simulink subsystem "OneAxleTrailer"  (R2023a)
settings: Solver=VariableStepAuto  StartTime=0.0  StopTime=10.0  RelTol=1e-3
undefined symbols (not defined in the file): PlntTraCGHgtAxl, PlntTraDstCGMiddleAxl, PlntTraHtchCxy, PlntTraHtchCz, PlntTraHtchF0z, PlntTraHtchKxy, PlntTraHtchKz, PlntTraInitLatPos, PlntTraInitLatVel, PlntTraInitLongPos, PlntTraInitLongVel, PlntTraInitPitchAng, PlntTraInitPitchRate, PlntTraInitRollAng, PlntTraInitRollRate, PlntTraInitVertPos, PlntTraInitVertVel, PlntTraInitYawAng, PlntTraInitYawRate, PlntTraMass, PlntTraNumWhlFrntAxl, PlntTraPitchMomentInertia, PlntTraRollMomentInertia, PlntTraTrckWdth, PlntTraYawMomentInertia
libraries: autolibutils x7, sharedtransform x4, vehdynlibeom x2, vehdynlibsuspension x1, matrix_library x1
(part 1 of 2)
settings Model: ModifiedByFormat=The MathWorks, Inc.  Creator=The MathWorks, Inc.  LastModifiedBy=The MathWorks, Inc.
settings SolverCC: MaxZcPerStep=1
settings OptimizationCC: ReuseModelBlockBuffer=off
settings DebuggingCC: UnconnectedInputMsg=warning  UnconnectedOutputMsg=warning  UnconnectedLineMsg=warning
settings ModelReferenceCC: EnableRefExpFcnMdlSchedulingChecks=on
settings RTWCC: DLArmComputeVersion=19.05

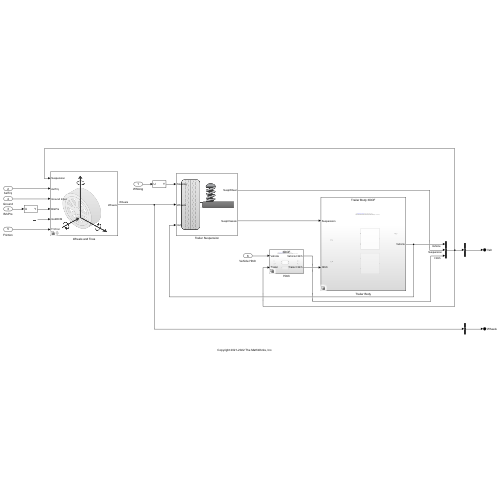
[thumbnail: Simulink's stored preview of the top-level diagram]
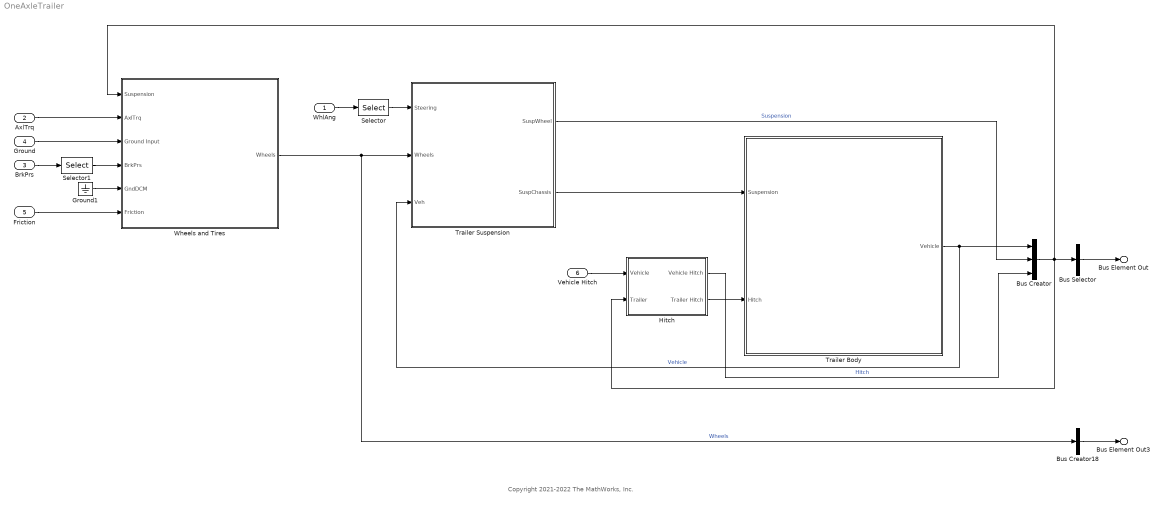
== system OneAxleTrailer ==
  note: Copyright 2021-2022 The MathWorks, Inc.
  WhlAng : Inport
  AxlTrq : Inport  Port=2
  BrkPrs : Inport  Port=3
  Ground : Inport  Port=4
  Friction : Inport  Port=5
  Vehicle Hitch : Inport  Port=6
  Bus Creator : BusCreator  Inputs=3
  Bus Creator18 : BusCreator  Inputs=1
  Bus Selector : BusSelector  OutputSignals=Vehicle.InertFrm,Vehicle.BdyFrm,Hitch  OutputAsBus=on
  Ground1 : Ground
  Hitch : Subsystem  Variant=on  VariantControlMode=label  LabelModeActiveChoice=0
  Selector : Selector  IndexOptions=Index vector (dialog)  Indices=[1 2]  OutputSizes=1
  Selector1 : Selector  IndexOptions=Index vector (dialog)  Indices=[1 2]  OutputSizes=1
  Trailer Body : Subsystem  Variant=on  VariantControlMode=label  LabelModeActiveChoice=0
  Trailer Suspension : Subsystem
      mask Display: image('suspsacoil.png')
  Wheels and Tires : Subsystem  Variant=on  VariantControlMode=label  VariantControl=Choice  LabelModeActiveChoice=MF Tires Longitudinal and Lateral
      mask Display: image('wheel3dof.png')
  Bus Element Out : Outport  PortName=Veh
  Bus Element Out3 : Outport  Port=2  PortName=Wheels
  wires:
  Trailer Suspension/1(SuspWheel) -> Bus Creator/2  "Suspension"
  Trailer Suspension/2(SuspChassis) -> Trailer Body/1(Suspension)
  Bus Creator18/1 -> Bus Element Out3/1
  Vehicle Hitch/1 -> Hitch/1(Vehicle)
  Bus Selector/1 -> Bus Element Out/1
  Hitch/1(Vehicle Hitch) -> Bus Creator/3  "Hitch"
  AxlTrq/1 -> Wheels and Tires/2(AxlTrq)
  Bus Creator/1 -> Hitch/2(Trailer), Bus Selector/1, Wheels and Tires/1(Suspension)
  Wheels and Tires/1(Wheels) -> Bus Creator18/1, Trailer Suspension/2(Wheels)  "Wheels"
  BrkPrs/1 -> Selector1/1
  WhlAng/1 -> Selector/1
  Friction/1 -> Wheels and Tires/6(Friction)
  Trailer Body/1(Vehicle) -> Bus Creator/1, Trailer Suspension/3(Veh)  "Vehicle"
  Hitch/2(Trailer Hitch) -> Trailer Body/2(Hitch)
  Selector/1 -> Trailer Suspension/1(Steering)
  Selector1/1 -> Wheels and Tires/4(BrkPrs)
  Ground/1 -> Wheels and Tires/3(Ground Input)
  Ground1/1 -> Wheels and Tires/5(GndDCM)

== system OneAxleTrailer/Hitch ==
  note: 1) Add Subsystem or Model blocks as valid variant choices.
      | 2) You cannot connect blocks at this level. At simulation, connectivity is automatically
      | determined, based on the active variant and port name matching.
  Vehicle : Inport
  Trailer : Inport  Port=2
  3DOF : Subsystem  VariantControl=0
  6DOF : Subsystem  VariantControl=1
  Vehicle Hitch : Outport
  Trailer Hitch : Outport  Port=2

== system OneAxleTrailer/Trailer Body ==
  note: 1) Add Subsystem or Model blocks as valid variant choices.
      | 2) You cannot connect blocks at this level. At simulation, connectivity is automatically
      | determined, based on the active variant and port name matching.
  Suspension : Inport
  Hitch : Inport  Port=2
  Trailer Body 3DOF : Subsystem  VariantControl=0
  Trailer Body 6DOF : Subsystem  VariantControl=1
  Vehicle : Outport

== system OneAxleTrailer/Trailer Suspension ==
  Steering : Inport
  Wheels : Inport  Port=2
  Veh : Inport  Port=3
  Bus Creator : BusCreator  Inputs=2
  Solid Axle Suspension : Subsystem  VariantControl=MacPherson Front Suspension Solid Axle Rear Suspension
      mask Display: image('suspsacoil.png');
  Susp2Wheel : Subsystem
  Wheel2Susp : Subsystem
  SuspWheel : Outport
  SuspChassis : Outport  Port=2
  wires:
  Solid Axle Suspension/1(Suspension) -> Susp2Wheel/1(Susp), Bus Creator/1  "SuspChassis"
  Wheel2Susp/1(Wheels2Susp) -> Solid Axle Suspension/3(Wheels), Susp2Wheel/2(WheelSusp)
  Susp2Wheel/1(SuspWheel) -> SuspWheel/1, Bus Creator/2, Wheel2Susp/3(SuspWheel)  "SuspWheel"
  Wheels/1 -> Wheel2Susp/2(Wheels)
  Bus Creator/1 -> SuspChassis/1
  Veh/1 -> Wheel2Susp/1(Veh), Solid Axle Suspension/2(Vehicle)
  Steering/1 -> Solid Axle Suspension/1(Steer)

== system OneAxleTrailer/Wheels and Tires ==
  Suspension : Inport
  AxlTrq : Inport  Port=2
  Ground Input : Inport  Port=3
  BrkPrs : Inport  Port=4
  GndDCM : Inport  Port=5
  Friction : Inport  Port=6
  Combined Slip Tires Longitudinal : Subsystem  VariantControl=Combined Slip Tires Longitudinal  ReferencedSubsystem=CombinedSlipTrailerTiresLongitudinal
  Fiala Tires Longitudinal and Lateral : Subsystem  VariantControl=Fiala Tires Longitudinal and Lateral  ReferencedSubsystem=FialaTrailerTires
  MF Tires Longitudinal : Subsystem  VariantControl=MF Tires Longitudinal  ReferencedSubsystem=MFTrailerTiresLongitudinal
  MF Tires Longitudinal and Lateral : Subsystem  VariantControl=MF Tires Longitudinal and Lateral  ReferencedSubsystem=MFTrailerTires
  Wheels : Outport

== system OneAxleTrailer/Hitch/3DOF ==
  Vehicle : Inport
  Trailer : Inport  Port=2
  Bus Selector : BusSelector  OutputSignals=InertFrm.Hitch.Disp.X,InertFrm.Hitch.Disp.Y,InertFrm.Cg.Ang.psi,InertFrm.Hitch.Vel.Xdot,InertFrm.Hitch.Vel.Ydot
  Bus Selector1 : BusSelector  OutputSignals=Vehicle.InertFrm.HitchF.Disp.X,Vehicle.InertFrm.HitchF.Disp.Y,Vehicle.InertFrm.Cg.Ang.psi,Vehicle.BdyFrm.Forces.HitchF.Fz,Vehicle.InertFrm.HitchF.Vel.Xdot,Vehicle.InertFrm.HitchF.Vel.Ydot
  Mux : Mux  Inputs=6
  Mux1 : Mux  Inputs=6
  Subsystem3 : Subsystem
  Vehicle Hitch : Outport
  Trailer Hitch : Outport  Port=2
  wires:
  Subsystem3/6(Vehicle Mhz) -> Mux1/6
  Subsystem3/5(Vehicle Mhy) -> Mux1/5
  Subsystem3/4(Vehicle Mhx) -> Mux1/4
  Subsystem3/12(Trailer Mhz) -> Mux/6
  Subsystem3/11(Trailer Mhy) -> Mux/5
  Subsystem3/10(Trailer Mhx) -> Mux/4
  Bus Selector1/6 -> Subsystem3/11(Trailer Ydot)  "<Ydot>"
  Bus Selector1/5 -> Subsystem3/10(Trailer Xdot)  "<Xdot>"
  Bus Selector/5 -> Subsystem3/5(Vehicle Ydot)  "<Ydot>"
  Bus Selector/4 -> Subsystem3/4(Vehicle Xdot)  "<Xdot>"
  Subsystem3/8(Trailer Fy) -> Mux/2
  Subsystem3/7(Trailer Fx) -> Mux/1
  Subsystem3/3(Vehicle Fz) -> Mux1/3
  Subsystem3/2(Vehicle Fy) -> Mux1/2
  Subsystem3/1(Vehicle Fx) -> Mux1/1
  Bus Selector1/3 -> Subsystem3/8(Trailer psi)  "<psi>"
  Bus Selector1/4 -> Subsystem3/9(Trailer Fz)  "<Fz>"
  Bus Selector1/2 -> Subsystem3/7(Trailer Y)  "<Y>"
  Bus Selector1/1 -> Subsystem3/6(Trailer X)  "<X>"
  Bus Selector/3 -> Subsystem3/3(Vehicle psi)  "<psi>"
  Bus Selector/2 -> Subsystem3/2(Vehicle Y)  "<Y>"
  Bus Selector/1 -> Subsystem3/1(Vehicle X)  "<X>"
  Trailer/1 -> Bus Selector1/1
  Mux/1 -> Trailer Hitch/1
  Vehicle/1 -> Bus Selector/1
  Mux1/1 -> Vehicle Hitch/1
  Subsystem3/9(Trailer FzOut) -> Mux/3

== system OneAxleTrailer/Hitch/6DOF ==
  Vehicle : Inport
  Trailer : Inport  Port=2
  Bus Selector : BusSelector  OutputSignals=InertFrm.Hitch.Disp.X,InertFrm.Hitch.Disp.Y,InertFrm.Hitch.Disp.Z,InertFrm.Hitch.Vel.Xdot,InertFrm.Hitch.Vel.Ydot,InertFrm.Hitch.Vel.Zdot,InertFrm.Cg.Ang.psi
  Bus Selector1 : BusSelector  OutputSignals=Vehicle.InertFrm.HitchF.Disp.X,Vehicle.InertFrm.HitchF.Disp.Y,Vehicle.InertFrm.HitchF.Disp.Z,Vehicle.InertFrm.HitchF.Vel.Xdot,Vehicle.InertFrm.HitchF.Vel.Ydot,Vehicle.InertFrm.HitchF.Vel.Zdot,Vehicle.InertFrm.Cg.Ang.psi
  Mux : Mux  Inputs=6
  Mux1 : Mux  Inputs=6
  Subsystem3 : Subsystem
  Vehicle Hitch : Outport
  Trailer Hitch : Outport  Port=2
  wires:
  Subsystem3/6(Vehicle Mhz) -> Mux1/6
  Subsystem3/5(Vehicle Mhy) -> Mux1/5
  Subsystem3/4(Vehicle Mhx) -> Mux1/4
  Subsystem3/12(Trailer Mhz) -> Mux/6
  Subsystem3/11(Trailer Mhy) -> Mux/5
  Subsystem3/10(Trailer Mhx) -> Mux/4
  Bus Selector/5 -> Subsystem3/5(Vehicle Ydot)  "<Ydot>"
  Bus Selector/4 -> Subsystem3/4(Vehicle Xdot)  "<Xdot>"
  Bus Selector1/4 -> Subsystem3/11(Trailer Xdot)  "<Xdot>"
  Bus Selector1/5 -> Subsystem3/12(Trailer Ydot)  "<Ydot>"
  Bus Selector1/6 -> Subsystem3/13(Trailer Zdot)  "<Zdot>"
  Bus Selector/6 -> Subsystem3/6(Vehicle Zdot)  "<Zdot>"
  Bus Selector/3 -> Subsystem3/3(Vehicle Z)  "<Z>"
  Bus Selector1/3 -> Subsystem3/10(Trailer Z)  "<Z>"
  Subsystem3/8(Trailer Fy) -> Mux/2
  Subsystem3/7(Trailer Fx) -> Mux/1
  Subsystem3/3(Vehicle Fz) -> Mux1/3
  Subsystem3/2(Vehicle Fy) -> Mux1/2
  Subsystem3/1(Vehicle Fx) -> Mux1/1
  Bus Selector1/7 -> Subsystem3/14(Trailer psi)  "<psi>"
  Bus Selector1/2 -> Subsystem3/9(Trailer Y)  "<Y>"
  Bus Selector1/1 -> Subsystem3/8(Trailer X)  "<X>"
  Bus Selector/7 -> Subsystem3/7(Vehicle psi)  "<psi>"
  Bus Selector/2 -> Subsystem3/2(Vehicle Y)  "<Y>"
  Bus Selector/1 -> Subsystem3/1(Vehicle X)  "<X>"
  Trailer/1 -> Bus Selector1/1
  Mux/1 -> Trailer Hitch/1
  Vehicle/1 -> Bus Selector/1
  Mux1/1 -> Vehicle Hitch/1
  Subsystem3/9(Trailer Fz) -> Mux/3

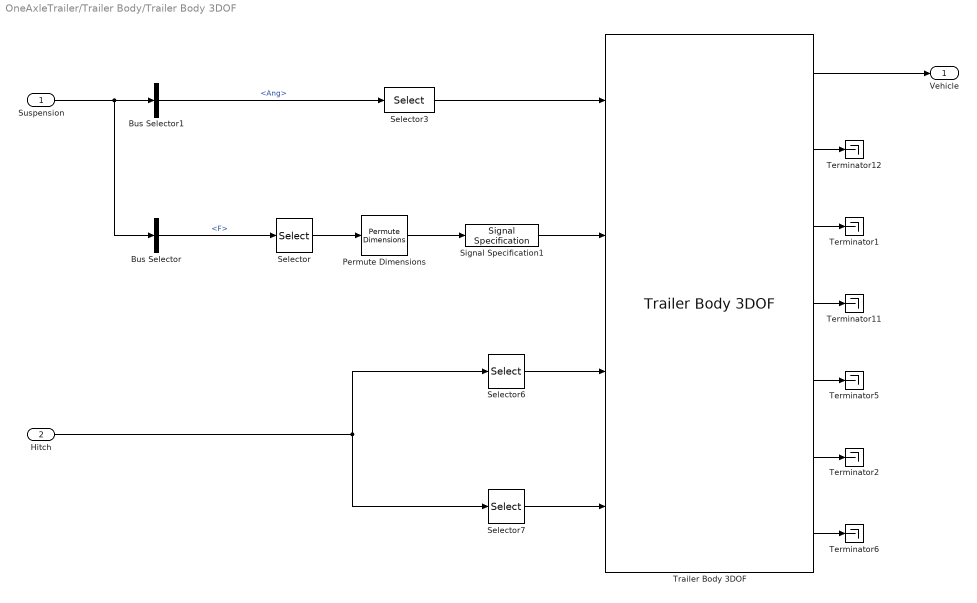
== system OneAxleTrailer/Trailer Body/Trailer Body 3DOF ==
  Suspension : Inport
  Hitch : Inport  Port=2
  Bus Selector : BusSelector  OutputSignals=SuspChassis.Veh.F
  Bus Selector1 : BusSelector  OutputSignals=SuspChassis.Whl.Ang
  Permute Dimensions : PermuteDimensions
  Selector : Selector  NumberOfDimensions=2  InputPortWidth=3  IndexOptions=Index vector (dialog),Index vector (dialog)  Indices=[1 2],[1 2]  OutputSizes=1,1
  Selector3 : Selector  NumberOfDimensions=2  InputPortWidth=6  IndexOptions=Index vector (dialog),Index vector (dialog)  Indices=3,[1 2]  OutputSizes=1,1
  Selector6 : Selector  InputPortWidth=6  IndexOptions=Index vector (dialog)  Indices=[1 2 3]  OutputSizes=1
  Selector7 : Selector  InputPortWidth=6  IndexOptions=Index vector (dialog)  Indices=[4 5 6]  OutputSizes=1
  Signal Specification1 : SignalSpecification  Unit=N
  Terminator{1..2,5..6,11..12} (6 alike) : Terminator
  Trailer Body 3DOF : vehdynlibeom/Trailer Body 3DOF  trackMode=Dual 1-axle  inputMode=External forces  frontSteerMode=on  middleSteerMode=off  rearSteerMode=off  windMode=off  muMode=off  extFMode=off  extMMode=off  FhtchFMode=on  FhtchMMode=on  RhtchFMode=off  RhtchMMode=off  extXo=off  extpsio=off  extxdoto=off  extro=off  extYo=off  extTamb=off  extydoto=off  aMode=2  NF=PlntTraNumWhlFrntAxl  NM=PlntTraNumWhlMiddleAxl  NR=PlntTraNumWhlRearAxl  m=PlntTraMass  a=PlntTraDstCGFrntAxl  b=PlntTraDstCGMiddleAxl  c=PlntTraDstCGRearAxl  h=PlntTraCGHgtAxl  dh_f=PlntTraHtchDstFrnt  hh_f=PlntTraHtchHgtAxlFrnt  dh_r=7.5  hh_r=0.6  X_o=PlntTraInitLongPos  xdot_o=PlntTraInitLongVel  Lcpm=4.5  CalphaMode=off  sigmaMode=on  d=0  hl_f=0  hl_r=0  w_f=PlntTraTrckWdth  w_m=PlntTraTrckWdth  w_r=PlntTraTrckWdth  Cy_f=12e3  Cy_m=11e3  Cy_r=11e3  sigma_f=.1  sigma_m=.1  sigma_r=.1  alpha_f_brk=[-.1 .1]  Cy_f_data=[-9e3 9e3]  alpha_m_brk=[-.1 .1]  Cy_m_data=[-9e3 9e3]  alpha_r_brk=[-.1 .1]  Cy_r_data=[-9e3 9e3]  Y_o=PlntTraInitLatPos  ydot_o=PlntTraInitLatVel  Izz=PlntTraYawMomentInertia  psi_o=PlntTraInitYawAng  r_o=PlntTraInitYawRate  Af=PlntTraAeroFrntArea  Cd=PlntTraAeroDragCff  Cl=PlntTraAeroLiftCff  Cpm=PlntTraAeroPitchCff  beta_w=[0:0.01:0.3]  Cs=[0:0.03:0.9]*0  Cym=[0:0.01:0.3]*0  Pabs=101325  Tair=273  g=9.81  mu=1  xdot_tol=.01  Fznom=5000  Fxtire_sat=7e4  Fytire_sat=7e4  longOff=0  latOff=0  vertOff=0  wrapAng=off
  Vehicle : Outport
  wires:
  Selector7/1 -> Trailer Body 3DOF/4
  Hitch/1 -> Selector6/1, Selector7/1
  Selector6/1 -> Trailer Body 3DOF/3
  Trailer Body 3DOF/4 -> Terminator11/1
  Bus Selector/1 -> Selector/1  "<F>"
  Trailer Body 3DOF/1 -> Vehicle/1
  Selector/1 -> Permute Dimensions/1
  Permute Dimensions/1 -> Signal Specification1/1
  Trailer Body 3DOF/5 -> Terminator5/1
  Selector3/1 -> Trailer Body 3DOF/1
  Signal Specification1/1 -> Trailer Body 3DOF/2
  Bus Selector1/1 -> Selector3/1  "<Ang>"
  Trailer Body 3DOF/3 -> Terminator1/1
  Trailer Body 3DOF/2 -> Terminator12/1
  Trailer Body 3DOF/7 -> Terminator6/1
  Trailer Body 3DOF/6 -> Terminator2/1
  Suspension/1 -> Bus Selector1/1, Bus Selector/1

== system OneAxleTrailer/Trailer Body/Trailer Body 6DOF ==
  Suspension : Inport
  Hitch : Inport  Port=2
  Bus Selector3 : BusSelector  OutputSignals=SuspChassis.Veh.F,SuspChassis.Veh.M
  Constant1 : Constant  Value=zeros(3,1)  SampleTime=-1
  Constant2 : Constant  Value=zeros(3,1)  SampleTime=-1
  Constant3 : Constant  Value=zeros(3,1)  SampleTime=-1
  Selector6 : Selector  InputPortWidth=6  IndexOptions=Index vector (dialog)  Indices=[1 2 3]  OutputSizes=1
  Selector7 : Selector  InputPortWidth=6  IndexOptions=Index vector (dialog)  Indices=[4 5 6]  OutputSizes=1
  Terminator{,1..5} (6 alike) : Terminator
  Trailer Body 6DOF : vehdynlibeom/Trailer Body 6DOF  axleMode=1  extPos=on  extVel=on  extEuler=on  extRotRate=on  htchFMode_f=on  htchMMode_f=on  htchFMode_r=off  htchMMode_r=off  m=PlntTraMass  a=PlntTraDstCGFrntAxl  b=PlntTraDstCGMiddleAxl  c=PlntTraDstCGRearAxl  d=0  h=PlntTraCGHgtAxl  dh_f=PlntTraHtchDstFrnt  hl_f=0  hh_f=PlntTraHtchHgtAxlFrnt  dh_r=1  hl_r=0  hh_r=0.1  Xe_o=[PlntTraInitLongPos,PlntTraInitLatPos,PlntTraInitVertPos]  xbdot_o=[PlntTraInitLongVel,PlntTraInitLatVel,PlntTraInitVertVel]  eul_o=[PlntTraInitRollAng,PlntTraInitPitchAng,PlntTraInitYawAng]  p_o=[PlntTraInitRollRate,PlntTraInitPitchRate,PlntTraInitYawRate]  Iveh=[PlntTraRollMomentInertia 0 0; 0 PlntTraPitchMomentInertia 0; 0 0 PlntTraYawMomentInertia]  w_f=PlntTraTrckWdth  w_m=PlntTraTrckWdth  w_r=PlntTraTrckWdth  z1m=0  z1R=[-.25,.125,.15]  z1I=[1.4,-.2,.1;-.2,1.4,.1;.1,.1,2.25].*0  z2m=0  z2R=[1.4,0,.8]  z2I=[1.4,-.2,.1;-.2,1.4,.1;.1,.1,2.25].*0  z3m=0  z3R=[.75,-.5,.4]  z3I=[5,-.1,-2;-2,9,.1;-.1,.1,6].*0  z4m=0  z4R=[.75,.5,.4]  z4I=[5,-.1,-2;-2,9,.1;-.1,.1,6].*0  z5m=0  z5R=[1.25,-.5,.4]  z5I=[5,-.1,-2;-2,9,.1;-.1,.1,6].*0  z6m=0  z6R=[1.25,-.5,.4]  z6I=[5,-.1,-2;-2,9,.1;-.1,.1,6].*0  z7m=0  z7R=[2,0,.25]  z7I=[1.4,-.2,.1;-.2,1.4,.1;.1,.1,2.25].*0  Af=PlntTraAeroFrntArea  Cd=PlntTraAeroDragCff  Cl=PlntTraAeroLiftCff  Cpm=PlntTraAeroPitchCff  beta_w=[0:0.01:0.3]  Cs=[0:0.03:0.9]  Cym=[0:0.01:0.3]  Pabs=101325  extTamb=off  Tair=273  g=9.81  xdot_tol=.1  longOff=0  latOff=0  vertOff=0.0112  wrapAng=off  aMode=2
  Vehicle : Outport
  wires:
  Selector7/1 -> Trailer Body 6DOF/6
  Selector6/1 -> Trailer Body 6DOF/5
  Hitch/1 -> Selector6/1, Selector7/1
  Constant1/1 -> Trailer Body 6DOF/7
  Trailer Body 6DOF/1 -> Vehicle/1
  Trailer Body 6DOF/2 -> Terminator5/1
  Trailer Body 6DOF/3 -> Terminator4/1
  Trailer Body 6DOF/4 -> Terminator3/1
  Trailer Body 6DOF/5 -> Terminator2/1
  Trailer Body 6DOF/6 -> Terminator1/1
  Trailer Body 6DOF/7 -> Terminator/1
  Constant3/1 -> Trailer Body 6DOF/4
  Constant2/1 -> Trailer Body 6DOF/3
  Bus Selector3/1 -> Trailer Body 6DOF/1  "<F>"
  Bus Selector3/2 -> Trailer Body 6DOF/2  "<M>"
  Suspension/1 -> Bus Selector3/1

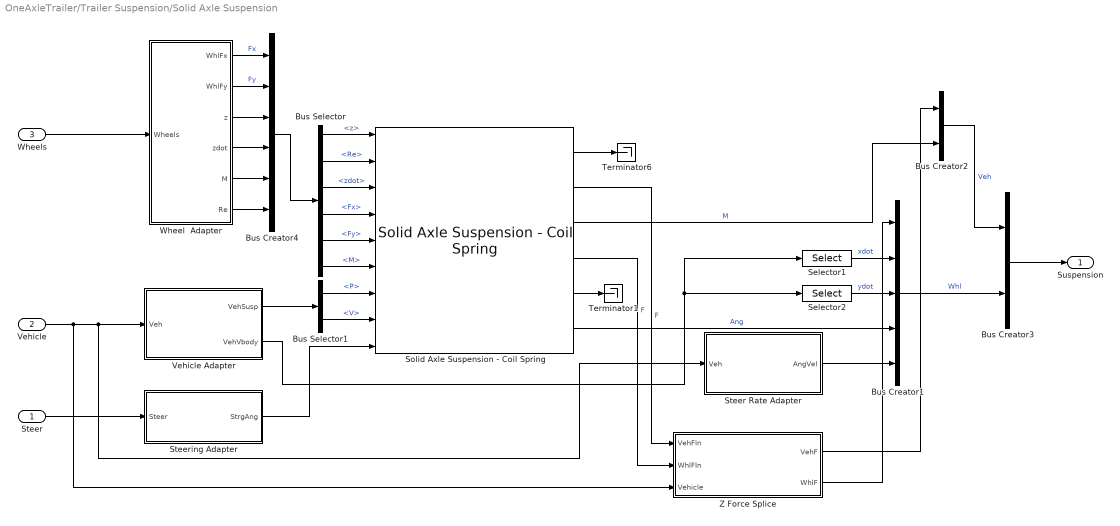
== system OneAxleTrailer/Trailer Suspension/Solid Axle Suspension ==
  Steer : Inport
  Vehicle : Inport  Port=2
  Wheels : Inport  Port=3
  Bus Creator1 : BusCreator  Inputs=5
  Bus Creator2 : BusCreator  Inputs=2
  Bus Creator3 : BusCreator  Inputs=2
  Bus Creator4 : BusCreator  Inputs=6
  Bus Selector : BusSelector  OutputSignals=z,Re,zdot,Fx,Fy,M
  Bus Selector1 : BusSelector  OutputSignals=P,V
  Selector1 : Selector  NumberOfDimensions=2  InputPortWidth=3  IndexOptions=Index vector (dialog),Select all  Indices=1,1  OutputSizes=1,1
  Selector2 : Selector  NumberOfDimensions=2  InputPortWidth=3  IndexOptions=Index vector (dialog),Select all  Indices=2,1  OutputSizes=1,1
  Solid Axle Suspension - Coil Spring : vehdynlibsuspension/Solid Axle Suspension - Coil Spring  NumAxl=1  NumWhlsByAxl=PlntTraNumWhlFrntAxl  StrgEnByAxl=1  WhlNumVec="[1  2]"  AxleNumVec="[1  1]"  SuspTypesByAxle=[1]  SuspImage=suspsacoil.png  AxlIxx=PlntTraAxlIxx  AxlM=PlntTraAxlM  TrackCoords=[zeros(1,2);PlntTraTrckWdth*[1 -1]/2;zeros(1,2)]  SuspCoords=[zeros(1,2);PlntTraTrckWdth*[1 -1]/2;zeros(1,2)]  KzWhlAxl=PlntTraKzWhlAxl  F0zWhlAxl=PlntTraF0zWhlAxl  CzWhlAxl=PlntTraCzWhlAxl  IdealSuspEn=on  IdealSuspAxles=[1]  Kz=PlntTraSuspKz  F0z=PlntTraSuspF0z  Cz=PlntTraSuspCz  Hmax=PlntTraSuspHmax  Toe=0  RollStrgSlp=0  ToeStrgSlp=0  Caster=0  CasterHslp=0  CasterStrgSlp=0  Camber=0  CamberHslp=0  CamberStrgSlp=0  StrgHgtSlp=0.1432  MappedSuspEn=off  MappedSuspAxles="[1  2]"  f_susp_axl_bp=[1 2]  f_susp_dz_bp=[-0.15 -0.14 -0.13 -0.12 -0.11 -0.10 -0.09 -0.08 -0.07 -0.06 -0.05 -0.04 -0.03 -0.02 -0.01 0.00 0.01 0.02 0.03 0.04 0.05 0.06 0.07 0.08 0.09 0.10 0.11 0.12 0.13 0.14 0.15]  f_susp_dzdot_bp=[-0.15 -0.14 -0.13 -0.12 -0.11 -0.10 -0.09 -0.08 -0.07 -0.06 -0.05 -0.04 -0.03 -0.02 -0.01 0.00 0.01 0.02 0.03 0.04 0.05 0.06 0.07 0.08 0.09 0.10 0.11 0.12 0.13 0.14 0.15]  f_susp_fmz=zeros(31,31,61,2,4)  f_susp_geom=zeros(31,61,2,3)  f_susp_strgdelta_bp=[-30,-29,-28,-27,-26,-25,-24,-23,-22,-21,-20,-19,-18,-17,-16,-15,-14,-13,-12,-11,-10,-9,-8,-7,-6,-5,-4,-3,-2,-1,0,1,2,3,4,5,6,7,8,9,10,11,12,13,14,15,16,17,18,19,20,21,22,23,24,25,26,27,28,29,30]
  Steer Rate Adapter : Subsystem
  Steering Adapter : Subsystem
  Terminator1 : Terminator
  Terminator6 : Terminator
  Vehicle Adapter : Subsystem
  Wheel  Adapter : Subsystem
  Z Force Splice : Subsystem  Variant=on  VariantControlMode=label  LabelModeActiveChoice=0
  Suspension : Outport
  wires:
  Bus Selector/5 -> Solid Axle Suspension - Coil Spring/5  "<Fy>"
  Vehicle/1 -> Z Force Splice/3(Vehicle), Steer Rate Adapter/1(Veh), Vehicle Adapter/1(Veh)
  Wheel  Adapter/2(WhlFy) -> Bus Creator4/2  "Fy"
  Solid Axle Suspension - Coil Spring/3 -> Bus Creator2/2  "M"
  Z Force Splice/1(VehF) -> Bus Creator2/1
  Vehicle Adapter/1(VehSusp) -> Bus Selector1/1
  Wheel  Adapter/1(WhlFx) -> Bus Creator4/1  "Fx"
  Vehicle Adapter/2(VehVbody) -> Selector1/1, Selector2/1
  Bus Selector/2 -> Solid Axle Suspension - Coil Spring/2  "<Re>"
  Wheel  Adapter/5(M) -> Bus Creator4/5
  Bus Selector1/2 -> Solid Axle Suspension - Coil Spring/8  "<V>"
  Selector1/1 -> Bus Creator1/2  "xdot"
  Solid Axle Suspension - Coil Spring/2 -> Z Force Splice/1(VehFIn)  "F"
  Bus Selector1/1 -> Solid Axle Suspension - Coil Spring/7  "<P>"
  Wheel  Adapter/3(z) -> Bus Creator4/3
  Steering Adapter/1(StrgAng) -> Solid Axle Suspension - Coil Spring/9
  Bus Selector/4 -> Solid Axle Suspension - Coil Spring/4  "<Fx>"
  Bus Selector/1 -> Solid Axle Suspension - Coil Spring/1  "<z>"
  Bus Creator1/1 -> Bus Creator3/2  "Whl"
  Solid Axle Suspension - Coil Spring/6 -> Bus Creator1/4  "Ang"
  Solid Axle Suspension - Coil Spring/4 -> Z Force Splice/2(WhlFIn)  "F"
  Solid Axle Suspension - Coil Spring/1 -> Terminator6/1
  Steer Rate Adapter/1(AngVel) -> Bus Creator1/5
  Selector2/1 -> Bus Creator1/3  "ydot"
  Z Force Splice/2(WhlF) -> Bus Creator1/1
  Solid Axle Suspension - Coil Spring/5 -> Terminator1/1
  Bus Selector/3 -> Solid Axle Suspension - Coil Spring/3  "<zdot>"
  Bus Creator3/1 -> Suspension/1
  Wheel  Adapter/6(Re) -> Bus Creator4/6
  Bus Creator4/1 -> Bus Selector/1
  Bus Creator2/1 -> Bus Creator3/1  "Veh"
  Wheel  Adapter/4(zdot) -> Bus Creator4/4
  Bus Selector/6 -> Solid Axle Suspension - Coil Spring/6  "<M>"
  Wheels/1 -> Wheel  Adapter/1(Wheels)
  Steer/1 -> Steering Adapter/1(Steer)

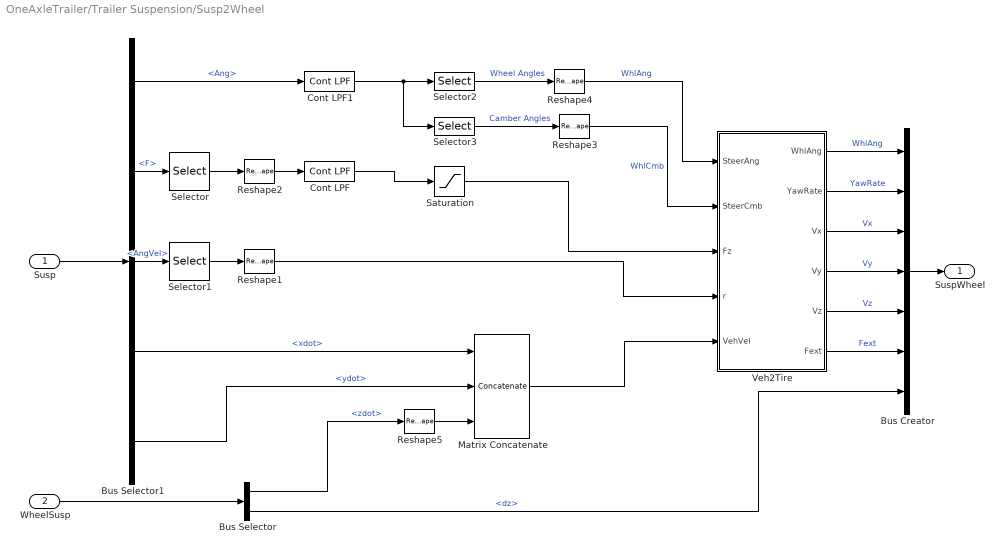
== system OneAxleTrailer/Trailer Suspension/Susp2Wheel ==
  Susp : Inport
  WheelSusp : Inport  Port=2
  Bus Creator : BusCreator  Inputs=7
  Bus Selector : BusSelector  OutputSignals=SuspFrame.zdot,SuspFrame.dz
  Bus Selector1 : BusSelector  OutputSignals=Whl.Ang,Whl.F,Whl.AngVel,Whl.xdot,Whl.ydot
  Cont LPF : autolibutils/Cont LPF  wc=100*2*pi  AbsoluteTolerance=auto  aMode=2
  Cont LPF1 : autolibutils/Cont LPF  wc=100*2*pi  AbsoluteTolerance=auto  aMode=2
  Matrix Concatenate : Concatenate  NumInputs=3  Mode=Multidimensional array
  Reshape{1..4} (4 alike) : Reshape
  Reshape5 : Reshape  OutputDimensionality=Row vector (2-D)
  Saturation : Saturate  UpperLimit=inf  LowerLimit=-10*9.81*2000  ZeroCross=off
  Selector : Selector  NumberOfDimensions=2  InputPortWidth=3  IndexOptions=Index vector (dialog),Select all  Indices=[3],1  OutputSizes=1,1
  Selector1 : Selector  NumberOfDimensions=2  InputPortWidth=1  IndexOptions=Index vector (dialog),Select all  Indices=[3],1  OutputSizes=1,1
  Selector2 : Selector  NumberOfDimensions=2  InputPortWidth=3  IndexOptions=Index vector (dialog),Select all  Indices=3,1  OutputSizes=1,1
  Selector3 : Selector  NumberOfDimensions=2  InputPortWidth=3  IndexOptions=Index vector (dialog),Select all  Indices=1,1  OutputSizes=1,1
  Veh2Tire : Subsystem
  SuspWheel : Outport
  wires:
  Bus Creator/1 -> SuspWheel/1
  Bus Selector/1 -> Reshape5/1  "<zdot>"
  Veh2Tire/3(Vx) -> Bus Creator/3  "Vx"
  Veh2Tire/4(Vy) -> Bus Creator/4  "Vy"
  Susp/1 -> Bus Selector1/1
  Veh2Tire/5(Vz) -> Bus Creator/5  "Vz"
  Bus Selector1/1 -> Cont LPF1/1  "<Ang>"
  Reshape5/1 -> Matrix Concatenate/3
  WheelSusp/1 -> Bus Selector/1
  Cont LPF/1 -> Saturation/1
  Selector/1 -> Reshape2/1
  Matrix Concatenate/1 -> Veh2Tire/5(VehVel)
  Saturation/1 -> Veh2Tire/3(Fz)
  Selector1/1 -> Reshape1/1
  Veh2Tire/6(Fext) -> Bus Creator/6  "Fext"
  Bus Selector1/5 -> Matrix Concatenate/2  "<ydot>"
  Bus Selector1/3 -> Selector1/1  "<AngVel>"
  Bus Selector1/4 -> Matrix Concatenate/1  "<xdot>"
  Reshape4/1 -> Veh2Tire/1(SteerAng)  "WhlAng"
  Veh2Tire/1(WhlAng) -> Bus Creator/1  "WhlAng"
  Reshape3/1 -> Veh2Tire/2(SteerCmb)  "WhlCmb"
  Selector3/1 -> Reshape3/1  "Camber Angles"
  Reshape2/1 -> Cont LPF/1
  Selector2/1 -> Reshape4/1  "Wheel Angles"
  Reshape1/1 -> Veh2Tire/4(r)
  Cont LPF1/1 -> Selector3/1, Selector2/1
  Bus Selector1/2 -> Selector/1  "<F>"
  Veh2Tire/2(YawRate) -> Bus Creator/2  "YawRate"
  Bus Selector/2 -> Bus Creator/7  "<dz>"

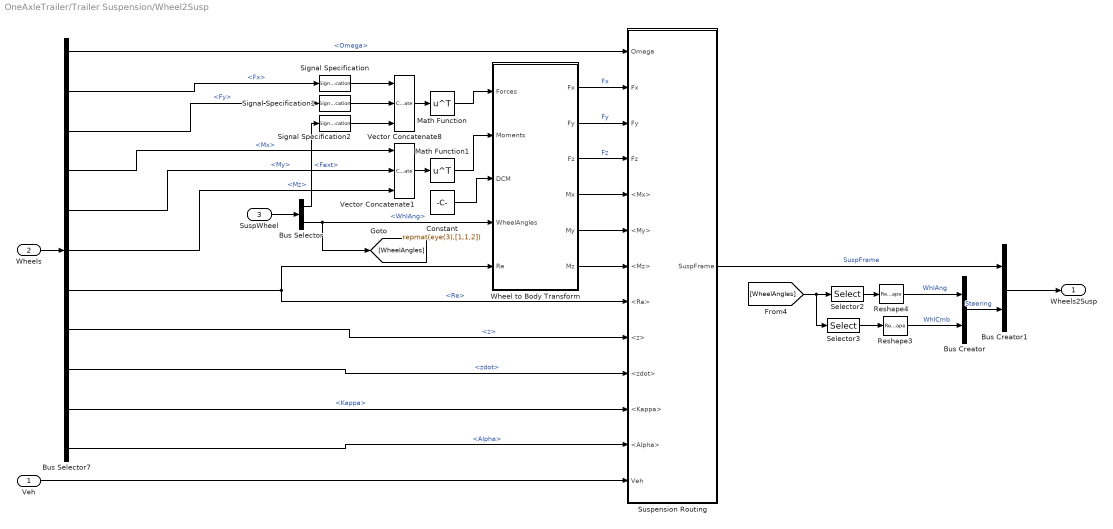
== system OneAxleTrailer/Trailer Suspension/Wheel2Susp ==
  Veh : Inport
  Wheels : Inport  Port=2
  SuspWheel : Inport  Port=3
  Bus Creator : BusCreator  Inputs=2
  Bus Creator1 : BusCreator  Inputs=2
  Bus Selector : BusSelector  OutputSignals=Fext,WhlAng
  Bus Selector7 : BusSelector  OutputSignals=Wheels.TireFrame.Omega,Wheels.TireFrame.Fx,Wheels.TireFrame.Fy,Wheels.TireFrame.Mx,Wheels.TireFrame.My,Wheels.TireFrame.Mz,Wheels.TireFrame.Re,Wheels.TireFrame.z,Wheels.TireFrame.zdot,Wheels.TireFrame.Kappa,Wheels.TireFrame.Alpha
  Constant : Constant  Value=repmat(eye(3),[1,1,2])
  Math Function : Math  Operator=transpose  SignedPower=on
  Math Function1 : Math  Operator=transpose  SignedPower=on
  Reshape3 : Reshape
  Reshape4 : Reshape
  Selector2 : Selector  NumberOfDimensions=2  InputPortWidth=3  IndexOptions=Index vector (dialog),Select all  Indices=3,1  OutputSizes=1,1
  Selector3 : Selector  NumberOfDimensions=2  InputPortWidth=3  IndexOptions=Index vector (dialog),Select all  Indices=1,1  OutputSizes=1,1
  Signal Specification : SignalSpecification  Dimensions=2
  Signal Specification1 : SignalSpecification  Dimensions=2
  Signal Specification2 : SignalSpecification  Dimensions=2
  Suspension Routing : Subsystem
  Vector Concatenate1 : Concatenate  NumInputs=3  Mode=Multidimensional array  ConcatenateDimension=2
  Vector Concatenate8 : Concatenate  NumInputs=3  Mode=Multidimensional array  ConcatenateDimension=2
  Wheel to Body Transform : Subsystem
  Wheels2Susp : Outport  VectorParamsAs1DForOutWhenUnconnected=off
  wires:
  Bus Selector7/11 -> Suspension Routing/12(<Alpha>)  "<Alpha>"
  Bus Selector7/10 -> Suspension Routing/11(<Kappa>)  "<Kappa>"
  Bus Selector7/9 -> Suspension Routing/10(<zdot>)  "<zdot>"
  Bus Selector7/8 -> Suspension Routing/9(<z>)  "<z>"
  Bus Selector7/7 -> Suspension Routing/8(<Re>), Wheel to Body Transform/5(Re)  "<Re>"
  Bus Selector7/6 -> Vector Concatenate1/3  "<Mz>"
  Bus Selector7/5 -> Vector Concatenate1/2  "<My>"
  Bus Selector7/4 -> Vector Concatenate1/1  "<Mx>"
  Bus Selector7/3 -> Signal Specification1/1  "<Fy>"
  Bus Selector7/2 -> Signal Specification/1  "<Fx>"
  Bus Selector7/1 -> Suspension Routing/1(Omega)  "<Omega>"
  Constant/1 -> Wheel to Body Transform/3(DCM)
  Math Function1/1 -> Wheel to Body Transform/2(Moments)
  Vector Concatenate1/1 -> Math Function1/1
  Wheel to Body Transform/6(Mz) -> Suspension Routing/7(<Mz>)
  Wheel to Body Transform/5(My) -> Suspension Routing/6(<My>)
  Wheel to Body Transform/4(Mx) -> Suspension Routing/5(<Mx>)
  Selector3/1 -> Reshape3/1
  [WheelAngles] -> Selector3/1, Selector2/1
  Selector2/1 -> Reshape4/1
  Signal Specification2/1 -> Vector Concatenate8/3
  Bus Selector/1 -> Signal Specification2/1  "<Fext>"
  SuspWheel/1 -> Bus Selector/1
  Wheel to Body Transform/2(Fy) -> Suspension Routing/3(Fy)  "Fy"
  Wheel to Body Transform/1(Fx) -> Suspension Routing/2(Fx)  "Fx"
  Vector Concatenate8/1 -> Math Function/1
  Math Function/1 -> Wheel to Body Transform/1(Forces)
  Wheels/1 -> Bus Selector7/1
  Bus Selector/2 -> Wheel to Body Transform/4(WheelAngles), [WheelAngles]  "<WhlAng>"
  Wheel to Body Transform/3(Fz) -> Suspension Routing/4(Fz)  "Fz"
  Reshape4/1 -> Bus Creator/1  "WhlAng"
  Bus Creator1/1 -> Wheels2Susp/1
  Suspension Routing/1(SuspFrame) -> Bus Creator1/1  "SuspFrame"
  Reshape3/1 -> Bus Creator/2  "WhlCmb"
  Bus Creator/1 -> Bus Creator1/2  "Steering"
  Veh/1 -> Suspension Routing/13(Veh)
  Signal Specification/1 -> Vector Concatenate8/1
  Signal Specification1/1 -> Vector Concatenate8/2

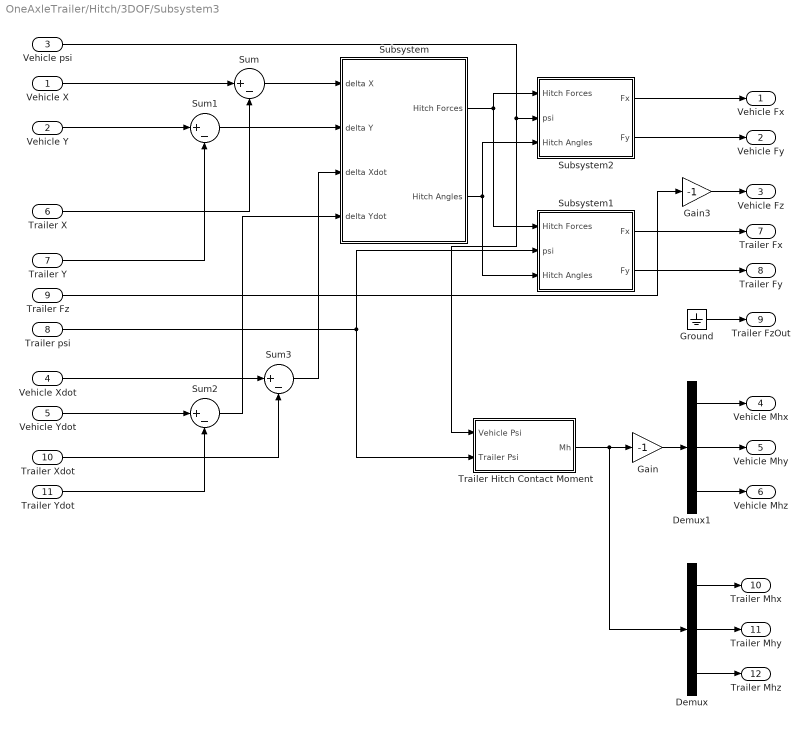
== system OneAxleTrailer/Hitch/3DOF/Subsystem3 ==
  Vehicle X : Inport
  Vehicle Y : Inport  Port=2
  Vehicle psi : Inport  Port=3
  Vehicle Xdot : Inport  Port=4
  Vehicle Ydot : Inport  Port=5
  Trailer X : Inport  Port=6
  Trailer Y : Inport  Port=7
  Trailer psi : Inport  Port=8
  Trailer Fz : Inport  Port=9
  Trailer Xdot : Inport  Port=10
  Trailer Ydot : Inport  Port=11
  Demux : Demux  Outputs=3
  Demux1 : Demux  Outputs=3
  Gain : Gain  Gain=-1
  Gain3 : Gain  Gain=-1
  Ground : Ground
  Subsystem : Subsystem
  Subsystem1 : Subsystem
  Subsystem2 : Subsystem
  Sum{,1..3} (4 alike) : Sum  Inputs=|+-
  Trailer Hitch Contact Moment : Subsystem
  Vehicle Fx : Outport
  Vehicle Fy : Outport  Port=2
  Vehicle Fz : Outport  Port=3
  Vehicle Mhx : Outport  Port=4
  Vehicle Mhy : Outport  Port=5
  Vehicle Mhz : Outport  Port=6
  Trailer Fx : Outport  Port=7
  Trailer Fy : Outport  Port=8
  Trailer FzOut : Outport  Port=9
  Trailer Mhx : Outport  Port=10
  Trailer Mhy : Outport  Port=11
  Trailer Mhz : Outport  Port=12
  wires:
  Ground/1 -> Trailer FzOut/1
  Demux/2 -> Trailer Mhy/1
  Gain/1 -> Demux1/1
  Trailer Hitch Contact Moment/1(Mh) -> Gain/1, Demux/1
  Demux/3 -> Trailer Mhz/1
  Demux1/3 -> Vehicle Mhz/1
  Demux/1 -> Trailer Mhx/1
  Demux1/1 -> Vehicle Mhx/1
  Demux1/2 -> Vehicle Mhy/1
  Sum2/1 -> Subsystem/4(delta Ydot)
  Sum3/1 -> Subsystem/3(delta Xdot)
  Vehicle Ydot/1 -> Sum2/1
  Vehicle Xdot/1 -> Sum3/1
  Trailer Ydot/1 -> Sum2/2
  Trailer Xdot/1 -> Sum3/2
  Trailer X/1 -> Sum/2
  Vehicle X/1 -> Sum/1
  Subsystem/1(Hitch Forces) -> Subsystem1/1(Hitch Forces), Subsystem2/1(Hitch Forces)
  Sum/1 -> Subsystem/1(delta X)
  Subsystem1/1(Fx) -> Trailer Fx/1
  Sum1/1 -> Subsystem/2(delta Y)
  Gain3/1 -> Vehicle Fz/1
  Subsystem1/2(Fy) -> Trailer Fy/1
  Trailer Y/1 -> Sum1/2
  Vehicle Y/1 -> Sum1/1
  Subsystem2/1(Fx) -> Vehicle Fx/1
  Subsystem2/2(Fy) -> Vehicle Fy/1
  Trailer psi/1 -> Trailer Hitch Contact Moment/2(Trailer Psi), Subsystem1/2(psi)
  Vehicle psi/1 -> Subsystem2/2(psi), Trailer Hitch Contact Moment/1(Vehicle Psi)
  Subsystem/2(Hitch Angles) -> Subsystem1/3(Hitch Angles), Subsystem2/3(Hitch Angles)
  Trailer Fz/1 -> Gain3/1

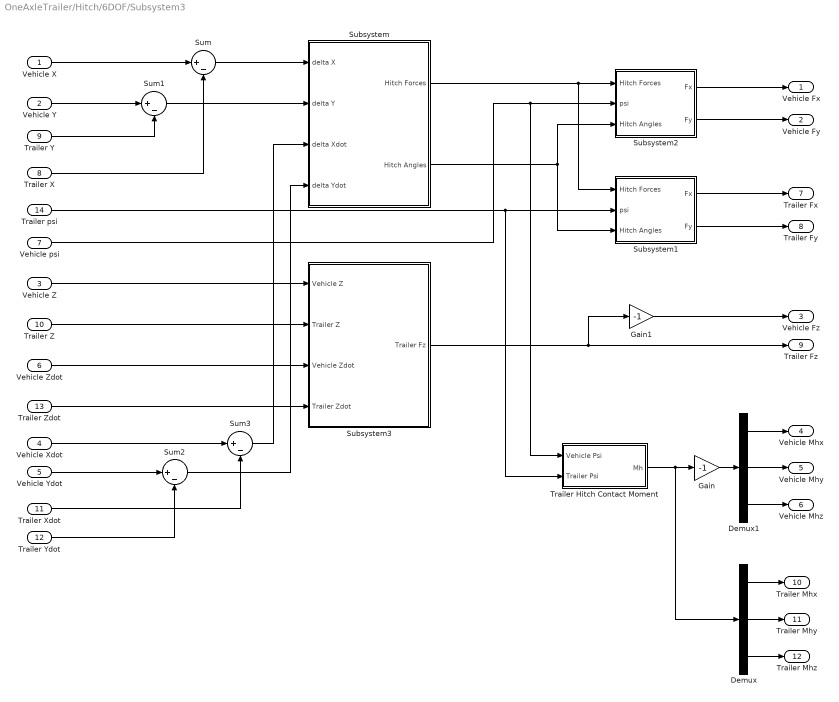
== system OneAxleTrailer/Hitch/6DOF/Subsystem3 ==
  Vehicle X : Inport
  Vehicle Y : Inport  Port=2
  Vehicle Z : Inport  Port=3
  Vehicle Xdot : Inport  Port=4
  Vehicle Ydot : Inport  Port=5
  Vehicle Zdot : Inport  Port=6
  Vehicle psi : Inport  Port=7
  Trailer X : Inport  Port=8
  Trailer Y : Inport  Port=9
  Trailer Z : Inport  Port=10
  Trailer Xdot : Inport  Port=11
  Trailer Ydot : Inport  Port=12
  Trailer Zdot : Inport  Port=13
  Trailer psi : Inport  Port=14
  Demux : Demux  Outputs=3
  Demux1 : Demux  Outputs=3
  Gain : Gain  Gain=-1
  Gain1 : Gain  Gain=-1
  Subsystem : Subsystem
  Subsystem1 : Subsystem
  Subsystem2 : Subsystem
  Subsystem3 : Subsystem
  Sum{,1..3} (4 alike) : Sum  Inputs=|+-
  Trailer Hitch Contact Moment : Subsystem
  Vehicle Fx : Outport
  Vehicle Fy : Outport  Port=2
  Vehicle Fz : Outport  Port=3
  Vehicle Mhx : Outport  Port=4
  Vehicle Mhy : Outport  Port=5
  Vehicle Mhz : Outport  Port=6
  Trailer Fx : Outport  Port=7
  Trailer Fy : Outport  Port=8
  Trailer Fz : Outport  Port=9
  Trailer Mhx : Outport  Port=10
  Trailer Mhy : Outport  Port=11
  Trailer Mhz : Outport  Port=12
  wires:
  Demux/3 -> Trailer Mhz/1
  Gain/1 -> Demux1/1
  Demux1/1 -> Vehicle Mhx/1
  Demux/2 -> Trailer Mhy/1
  Demux1/2 -> Vehicle Mhy/1
  Demux/1 -> Trailer Mhx/1
  Trailer Hitch Contact Moment/1(Mh) -> Gain/1, Demux/1
  Demux1/3 -> Vehicle Mhz/1
  Sum3/1 -> Subsystem/3(delta Xdot)
  Sum2/1 -> Subsystem/4(delta Ydot)
  Trailer Xdot/1 -> Sum3/2
  Vehicle Ydot/1 -> Sum2/1
  Vehicle Xdot/1 -> Sum3/1
  Trailer Ydot/1 -> Sum2/2
  Trailer Zdot/1 -> Subsystem3/4(Trailer Zdot)
  Vehicle Zdot/1 -> Subsystem3/3(Vehicle Zdot)
  Gain1/1 -> Vehicle Fz/1
  Trailer Z/1 -> Subsystem3/2(Trailer Z)
  Vehicle Z/1 -> Subsystem3/1(Vehicle Z)
  Subsystem1/2(Fy) -> Trailer Fy/1
  Subsystem1/1(Fx) -> Trailer Fx/1
  Subsystem2/2(Fy) -> Vehicle Fy/1
  Subsystem2/1(Fx) -> Vehicle Fx/1
  Subsystem3/1(Trailer Fz) -> Trailer Fz/1, Gain1/1
  Subsystem/2(Hitch Angles) -> Subsystem1/3(Hitch Angles), Subsystem2/3(Hitch Angles)
  Vehicle psi/1 -> Trailer Hitch Contact Moment/1(Vehicle Psi), Subsystem2/2(psi)
  Trailer psi/1 -> Trailer Hitch Contact Moment/2(Trailer Psi), Subsystem1/2(psi)
  Vehicle Y/1 -> Sum1/1
  Trailer X/1 -> Sum/2
  Trailer Y/1 -> Sum1/2
  Vehicle X/1 -> Sum/1
  Sum1/1 -> Subsystem/2(delta Y)
  Sum/1 -> Subsystem/1(delta X)
  Subsystem/1(Hitch Forces) -> Subsystem1/1(Hitch Forces), Subsystem2/1(Hitch Forces)

== system OneAxleTrailer/Trailer Suspension/Solid Axle Suspension/Steer Rate Adapter ==
  Veh : Inport
  Add : Sum
  Bus Selector3 : BusSelector  OutputSignals=BdyFrm.Cg.AngVel.r
  Constant : Constant  Value=zeros(1,2)  SampleTime=-1
  Matrix Concatenate : Concatenate  NumInputs=3  Mode=Multidimensional array
  Matrix Concatenate1 : Concatenate  NumInputs=3  Mode=Multidimensional array
  Mux : Mux  Inputs=2
  Reshape2 : Reshape  OutputDimensionality=Row vector (2-D)
  Reshape3 : Reshape  OutputDimensionality=Row vector (2-D)
  Reshape4 : Reshape  OutputDimensionality=Row vector (2-D)
  SteerRates : Constant  Value=zeros(1,2)  SampleTime=-1
  AngVel : Outport  VectorParamsAs1DForOutWhenUnconnected=off
  wires:
  Reshape2/1 -> Matrix Concatenate1/1, Matrix Concatenate1/3, Matrix Concatenate1/2
  Constant/1 -> Reshape3/1
  Mux/1 -> Reshape4/1
  Bus Selector3/1 -> Mux/2, Mux/1  "<r>"
  Matrix Concatenate/1 -> Add/2
  SteerRates/1 -> Reshape2/1
  Reshape4/1 -> Matrix Concatenate/3
  Reshape3/1 -> Matrix Concatenate/2, Matrix Concatenate/1
  Matrix Concatenate1/1 -> Add/1
  Veh/1 -> Bus Selector3/1
  Add/1 -> AngVel/1  "AngVel"

== system OneAxleTrailer/Trailer Suspension/Solid Axle Suspension/Steering Adapter ==
  Steer : Inport
  Reshape1 : Reshape  OutputDimensionality=Row vector (2-D)
  StrgAng : Outport  VectorParamsAs1DForOutWhenUnconnected=off
  wires:
  Reshape1/1 -> StrgAng/1
  Steer/1 -> Reshape1/1

== system OneAxleTrailer/Trailer Suspension/Solid Axle Suspension/Vehicle Adapter ==
  Veh : Inport
  Bus Creator3 : BusCreator  Inputs=2
  Bus Selector1 : BusSelector  OutputSignals=InertFrm.FrntAxl.Lft.Disp.X,InertFrm.FrntAxl.Lft.Disp.Y,InertFrm.FrntAxl.Lft.Disp.Z,InertFrm.FrntAxl.Rght.Disp.X,InertFrm.FrntAxl.Rght.Disp.Y,InertFrm.FrntAxl.Rght.Disp.Z
  Bus Selector2 : BusSelector  OutputSignals=BdyFrm.FrntAxl.Lft.Vel.xdot,BdyFrm.FrntAxl.Lft.Vel.ydot,BdyFrm.FrntAxl.Lft.Vel.zdot,BdyFrm.FrntAxl.Rght.Vel.xdot,BdyFrm.FrntAxl.Rght.Vel.ydot,BdyFrm.FrntAxl.Rght.Vel.zdot
  Bus Selector3 : BusSelector  OutputSignals=InertFrm.FrntAxl.Lft.Vel.Xdot,InertFrm.FrntAxl.Lft.Vel.Ydot,InertFrm.FrntAxl.Lft.Vel.Zdot,InertFrm.FrntAxl.Rght.Vel.Xdot,InertFrm.FrntAxl.Rght.Vel.Ydot,InertFrm.FrntAxl.Rght.Vel.Zdot
  Inertial Frame CG to Axle Offset : Constant  Value=[zeros(2,2);PlntTraCGHgtAxl*ones(1,2)]  SampleTime=-1
  Mux1 : Mux  Inputs=6
  Mux2 : Mux  Inputs=6
  Mux3 : Mux  Inputs=6
  Reshape : Reshape  OutputDimensionality=Customize  OutputDimensions=[3,2]
  Reshape1 : Reshape  OutputDimensionality=Customize  OutputDimensions=[3,2]
  Reshape2 : Reshape  OutputDimensionality=Customize  OutputDimensions=[3,2]
  Sum : Sum  Inputs=|+-
  VehSusp : Outport  VectorParamsAs1DForOutWhenUnconnected=off
  VehVbody : Outport  Port=2  VectorParamsAs1DForOutWhenUnconnected=off
  wires:
  Bus Selector2/6 -> Mux1/6  "<zdot>"
  Bus Selector2/5 -> Mux1/5  "<ydot>"
  Bus Selector2/4 -> Mux1/4  "<xdot>"
  Bus Selector2/3 -> Mux1/3  "<zdot>"
  Bus Selector2/2 -> Mux1/2  "<ydot>"
  Bus Selector2/1 -> Mux1/1  "<xdot>"
  Bus Selector3/6 -> Mux3/6  "<Zdot>"
  Bus Selector3/5 -> Mux3/5  "<Ydot>"
  Bus Selector3/4 -> Mux3/4  "<Xdot>"
  Bus Selector3/3 -> Mux3/3  "<Zdot>"
  Bus Selector3/2 -> Mux3/2  "<Ydot>"
  Bus Selector3/1 -> Mux3/1  "<Xdot>"
  Bus Selector1/6 -> Mux2/6  "<Z>"
  Bus Selector1/5 -> Mux2/5  "<Y>"
  Bus Selector1/1 -> Mux2/1  "<X>"
  Bus Selector1/4 -> Mux2/4  "<X>"
  Bus Selector1/2 -> Mux2/2  "<Y>"
  Bus Selector1/3 -> Mux2/3  "<Z>"
  Reshape1/1 -> Bus Creator3/2  "V"
  Mux3/1 -> Reshape1/1
  Sum/1 -> Bus Creator3/1  "P"
  Inertial Frame CG to Axle Offset/1 -> Sum/2
  Mux2/1 -> Reshape/1
  Mux1/1 -> Reshape2/1
  Reshape/1 -> Sum/1
  Bus Creator3/1 -> VehSusp/1  "Veh"
  Reshape2/1 -> VehVbody/1  "V"
  Veh/1 -> Bus Selector1/1, Bus Selector2/1, Bus Selector3/1

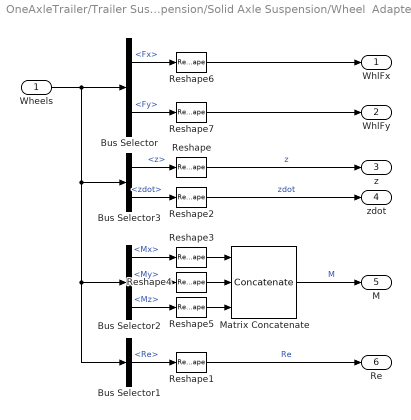
== system OneAxleTrailer/Trailer Suspension/Solid Axle Suspension/Wheel  Adapter ==
  Wheels : Inport
  Bus Selector : BusSelector  OutputSignals=SuspFrame.Fx,SuspFrame.Fy
  Bus Selector1 : BusSelector  OutputSignals=SuspFrame.Re
  Bus Selector2 : BusSelector  OutputSignals=SuspFrame.Mx,SuspFrame.My,SuspFrame.Mz
  Bus Selector3 : BusSelector  OutputSignals=SuspFrame.z,SuspFrame.zdot
  Matrix Concatenate : Concatenate  NumInputs=3  Mode=Multidimensional array
  Reshape{,1..7} (8 alike) : Reshape  OutputDimensionality=Row vector (2-D)
  WhlFx : Outport  VectorParamsAs1DForOutWhenUnconnected=off
  WhlFy : Outport  Port=2  VectorParamsAs1DForOutWhenUnconnected=off
  z : Outport  Port=3  VectorParamsAs1DForOutWhenUnconnected=off
  zdot : Outport  Port=4  VectorParamsAs1DForOutWhenUnconnected=off
  M : Outport  Port=5  VectorParamsAs1DForOutWhenUnconnected=off
  Re : Outport  Port=6  VectorParamsAs1DForOutWhenUnconnected=off
  wires:
  Reshape7/1 -> WhlFy/1
  Reshape6/1 -> WhlFx/1
  Bus Selector/1 -> Reshape6/1  "<Fx>"
  Bus Selector/2 -> Reshape7/1  "<Fy>"
  Bus Selector3/1 -> Reshape/1  "<z>"
  Wheels/1 -> Bus Selector1/1, Bus Selector2/1, Bus Selector3/1, Bus Selector/1
  Bus Selector3/2 -> Reshape2/1  "<zdot>"
  Reshape2/1 -> zdot/1  "zdot"
  Bus Selector1/1 -> Reshape1/1  "<Re>"
  Reshape1/1 -> Re/1  "Re"
  Bus Selector2/1 -> Reshape3/1  "<Mx>"
  Bus Selector2/2 -> Reshape4/1  "<My>"
  Bus Selector2/3 -> Reshape5/1  "<Mz>"
  Reshape3/1 -> Matrix Concatenate/1
  Reshape4/1 -> Matrix Concatenate/2
  Reshape5/1 -> Matrix Concatenate/3
  Matrix Concatenate/1 -> M/1  "M"
  Reshape/1 -> z/1  "z"

== system OneAxleTrailer/Trailer Suspension/Solid Axle Suspension/Z Force Splice ==
  note: 1) Add Subsystem or Model blocks as valid variant choices.
      | 2) You cannot connect blocks at this level. At simulation, connectivity is automatically
      | determined, based on the active variant and port name matching.
  VehFIn : Inport
  WhlFIn : Inport  Port=2
  Vehicle : Inport  Port=3
  Z Force Pass Through 6DOF : Subsystem  VariantControl=1
  Z Force Splice 3DOF : Subsystem  VariantControl=0
  VehF : Outport
  WhlF : Outport  Port=2

== system OneAxleTrailer/Trailer Suspension/Susp2Wheel/Veh2Tire ==
  SteerAng : Inport
  SteerCmb : Inport  Port=2
  Fz : Inport  Port=3
  r : Inport  Port=4
  VehVel : Inport  Port=5
  Reshape1 : Reshape
  Reshape2 : Reshape
  Reshape5 : Reshape
  Unary Minus : UnaryMinus
  Wheel Angles : Subsystem
  Wheel to Body Transform : Subsystem
  WhlAng : Outport  Unit=rad  VectorParamsAs1DForOutWhenUnconnected=off
  YawRate : Outport  Port=2  Unit=rad/s  VectorParamsAs1DForOutWhenUnconnected=off
  Vx : Outport  Port=3  Unit=m/s  VectorParamsAs1DForOutWhenUnconnected=off
  Vy : Outport  Port=4  Unit=m/s  VectorParamsAs1DForOutWhenUnconnected=off
  Vz : Outport  Port=5  Unit=m/s  VectorParamsAs1DForOutWhenUnconnected=off
  Fext : Outport  Port=6  Unit=N  VectorParamsAs1DForOutWhenUnconnected=off
  wires:
  Fz/1 -> Fext/1
  Wheel to Body Transform/1(xdotWheel) -> Reshape1/1  "Vx"
  Wheel to Body Transform/2(ydotWheel) -> Reshape2/1  "Vy"
  SteerAng/1 -> Wheel Angles/1(SteerAng)
  r/1 -> Unary Minus/1
  VehVel/1 -> Wheel to Body Transform/1(VelVeh)
  Wheel to Body Transform/3(zdotWheel) -> Reshape5/1  "Vz"
  Unary Minus/1 -> YawRate/1
  Wheel Angles/1("WhlAng ") -> WhlAng/1, Wheel to Body Transform/2(WheelAngles)
  Reshape1/1 -> Vx/1
  Reshape2/1 -> Vy/1
  Reshape5/1 -> Vz/1
  SteerCmb/1 -> Wheel Angles/2(SteerCmb)

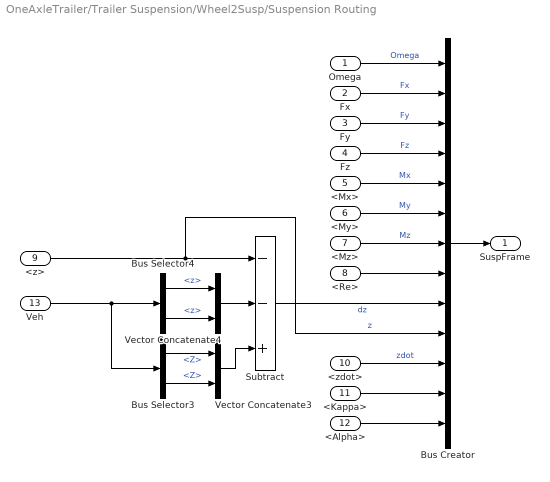
== system OneAxleTrailer/Trailer Suspension/Wheel2Susp/Suspension Routing ==
  Omega : Inport
  Fx : Inport  Port=2
  Fy : Inport  Port=3
  Fz : Inport  Port=4
  <Mx> : Inport  Port=5
  <My> : Inport  Port=6
  <Mz> : Inport  Port=7
  <Re> : Inport  Port=8
  <z> : Inport  Port=9
  <zdot> : Inport  Port=10
  <Kappa> : Inport  Port=11
  <Alpha> : Inport  Port=12
  Veh : Inport  Port=13
  Bus Creator : BusCreator  Inputs=13
  Bus Selector3 : BusSelector  OutputSignals=InertFrm.FrntAxl.Lft.Disp.Z,InertFrm.FrntAxl.Rght.Disp.Z
  Bus Selector4 : BusSelector  OutputSignals=BdyFrm.FrntAxl.Lft.Disp.z,BdyFrm.FrntAxl.Rght.Disp.z
  Subtract : Sum  Inputs=--+
  Vector Concatenate3 : Concatenate
  Vector Concatenate4 : Concatenate
  SuspFrame : Outport  VectorParamsAs1DForOutWhenUnconnected=off
  wires:
  <Re>/1 -> Bus Creator/8
  <z>/1 -> Subtract/1, Bus Creator/10  "z"
  Fz/1 -> Bus Creator/4  "Fz"
  <Mz>/1 -> Bus Creator/7  "Mz"
  <zdot>/1 -> Bus Creator/11  "zdot"
  Bus Creator/1 -> SuspFrame/1
  Fy/1 -> Bus Creator/3  "Fy"
  Omega/1 -> Bus Creator/1  "Omega"
  Fx/1 -> Bus Creator/2  "Fx"
  <Kappa>/1 -> Bus Creator/12
  <Mx>/1 -> Bus Creator/5  "Mx"
  <My>/1 -> Bus Creator/6  "My"
  <Alpha>/1 -> Bus Creator/13
  Veh/1 -> Bus Selector3/1, Bus Selector4/1
  Subtract/1 -> Bus Creator/9  "dz"
  Bus Selector4/1 -> Vector Concatenate4/1  "<z>"
  Bus Selector3/1 -> Vector Concatenate3/1  "<Z>"
  Vector Concatenate3/1 -> Subtract/3
  Vector Concatenate4/1 -> Subtract/2
  Bus Selector4/2 -> Vector Concatenate4/2  "<z>"
  Bus Selector3/2 -> Vector Concatenate3/2  "<Z>"

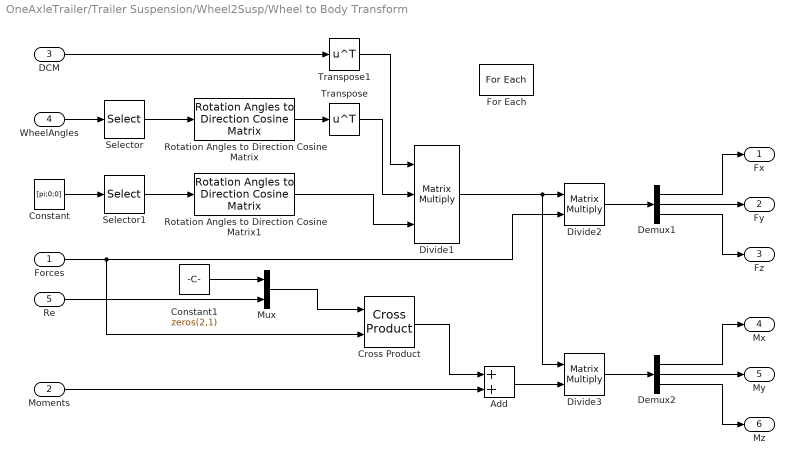
== system OneAxleTrailer/Trailer Suspension/Wheel2Susp/Wheel to Body Transform ==
  Forces : Inport  PortDimensions=[3,1]  Partition=on  PartitionDimension=2  PartitionWidth=1  PartitionOffset=0
  Moments : Inport  Port=2  PortDimensions=[3,1]  Partition=on  PartitionDimension=2  PartitionWidth=1  PartitionOffset=0
  DCM : Inport  Port=3  Partition=on  PartitionDimension=3  PartitionWidth=1  PartitionOffset=0
  WheelAngles : Inport  Port=4  Partition=on  PartitionDimension=2  PartitionWidth=1  PartitionOffset=0
  Re : Inport  Port=5  Partition=on  PartitionDimension=1  PartitionWidth=1  PartitionOffset=0
  Add : Sum
  Constant : Constant  Value=[pi;0;0]
  Constant1 : Constant  Value=zeros(2,1)
  Cross Product : matrix_library/Cross Product
  Demux1 : Demux  Outputs=3
  Demux2 : Demux  Outputs=3
  Divide1 : Product  Inputs=***  Multiplication=Matrix(*)
  Divide2 : Product  Inputs=**  Multiplication=Matrix(*)
  Divide3 : Product  Inputs=**  Multiplication=Matrix(*)
  For Each : ForEach  DisableCoverage=on
  Mux : Mux  Inputs=2
  Rotation Angles to Direction Cosine Matrix : sharedtransform/Rotation Angles to Direction Cosine Matrix  rotationOrder=ZYX  aMode=2
  Rotation Angles to Direction Cosine Matrix1 : sharedtransform/Rotation Angles to Direction Cosine Matrix  rotationOrder=ZYX  aMode=2
  Selector : Selector  InputPortWidth=3  IndexOptions=Index vector (dialog)  Indices=[3 2 1]  OutputSizes=1
  Selector1 : Selector  InputPortWidth=3  IndexOptions=Index vector (dialog)  Indices=[3 2 1]  OutputSizes=1
  Transpose : Math  Operator=transpose
  Transpose1 : Math  Operator=transpose
  Fx : Outport  ConcatenationDimension=1  VectorParamsAs1DForOutWhenUnconnected=off
  Fy : Outport  Port=2  ConcatenationDimension=1  VectorParamsAs1DForOutWhenUnconnected=off
  Fz : Outport  Port=3  ConcatenationDimension=1  VectorParamsAs1DForOutWhenUnconnected=off
  Mx : Outport  Port=4  ConcatenationDimension=1  VectorParamsAs1DForOutWhenUnconnected=off
  My : Outport  Port=5  ConcatenationDimension=1  VectorParamsAs1DForOutWhenUnconnected=off
  Mz : Outport  Port=6  ConcatenationDimension=1  VectorParamsAs1DForOutWhenUnconnected=off
  wires:
  Constant1/1 -> Mux/1
  Re/1 -> Mux/2
  Mux/1 -> Cross Product/1
  Cross Product/1 -> Add/1
  Add/1 -> Divide3/2
  Demux2/1 -> Mx/1
  Demux2/2 -> My/1
  Demux2/3 -> Mz/1
  Moments/1 -> Add/2
  Divide1/1 -> Divide2/1, Divide3/1
  Divide3/1 -> Demux2/1
  Divide2/1 -> Demux1/1
  Transpose1/1 -> Divide1/1
  DCM/1 -> Transpose1/1
  Transpose/1 -> Divide1/2
  Constant/1 -> Selector1/1
  Selector1/1 -> Rotation Angles to Direction Cosine Matrix1/1
  Rotation Angles to Direction Cosine Matrix1/1 -> Divide1/3
  Selector/1 -> Rotation Angles to Direction Cosine Matrix/1
  WheelAngles/1 -> Selector/1
  Forces/1 -> Cross Product/2, Divide2/2
  Rotation Angles to Direction Cosine Matrix/1 -> Transpose/1
  Demux1/3 -> Fz/1
  Demux1/2 -> Fy/1
  Demux1/1 -> Fx/1

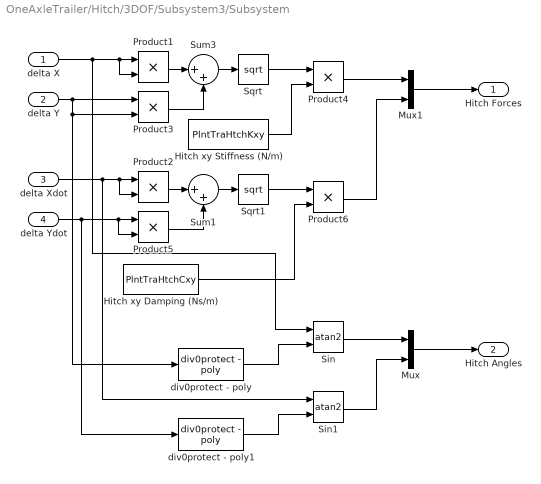
== system OneAxleTrailer/Hitch/3DOF/Subsystem3/Subsystem ==
  delta X : Inport
  delta Y : Inport  Port=2
  delta Xdot : Inport  Port=3
  delta Ydot : Inport  Port=4
  Hitch xy Damping (Ns/m) : Constant  Value=PlntTraHtchCxy  SampleTime=-1
  Hitch xy Stiffness (N/m) : Constant  Value=PlntTraHtchKxy  SampleTime=-1
  Mux : Mux  Inputs=2
  Mux1 : Mux  Inputs=2
  Product{1..6} (6 alike) : Product
  Sin : Trigonometry  Operator=atan2
  Sin1 : Trigonometry  Operator=atan2
  Sqrt : Sqrt
  Sqrt1 : Sqrt
  Sum1 : Sum  Inputs=|++
  Sum3 : Sum  Inputs=|++
  div0protect - poly : autolibutils/div0protect - poly  thresh=eps  ZeroCross=off  ZeroCross1=off  aMode=2
  div0protect - poly1 : autolibutils/div0protect - poly  thresh=eps  ZeroCross=off  ZeroCross1=off  aMode=2
  Hitch Forces : Outport
  Hitch Angles : Outport  Port=2
  wires:
  Product6/1 -> Mux1/2
  Mux1/1 -> Hitch Forces/1
  Sin1/1 -> Mux/2
  div0protect - poly1/1 -> Sin1/2
  Mux/1 -> Hitch Angles/1
  delta Ydot/1 -> Product5/2, Product5/1, div0protect - poly1/1
  Hitch xy Damping (Ns/m)/1 -> Product6/2
  delta Xdot/1 -> Product2/1, Product2/2, Sin1/1
  Sum1/1 -> Sqrt1/1
  Product2/1 -> Sum1/1
  Product5/1 -> Sum1/2
  Sqrt1/1 -> Product6/1
  Hitch xy Stiffness (N/m)/1 -> Product4/2
  Product4/1 -> Mux1/1
  Sqrt/1 -> Product4/1
  Product3/1 -> Sum3/2
  Product1/1 -> Sum3/1
  Sum3/1 -> Sqrt/1
  delta Y/1 -> div0protect - poly/1, Product3/2, Product3/1
  delta X/1 -> Product1/2, Product1/1, Sin/1
  Sin/1 -> Mux/1
  div0protect - poly/1 -> Sin/2

== system OneAxleTrailer/Hitch/3DOF/Subsystem3/Subsystem1 ==
  Hitch Forces : Inport
  psi : Inport  Port=2
  Hitch Angles : Inport  Port=3
  Cos : Trigonometry  Operator=cos
  Cos1 : Trigonometry
  Product1 : Product
  Product2 : Product
  Sum : Sum  Inputs=+
  Sum1 : Sum  Inputs=+
  Sum2 : Sum  Inputs=|++
  Fx : Outport
  Fy : Outport  Port=2
  wires:
  Sum1/1 -> Fx/1
  Sum/1 -> Fy/1
  Cos1/1 -> Product1/1
  Hitch Angles/1 -> Sum2/1
  Hitch Forces/1 -> Product2/2, Product1/2
  psi/1 -> Sum2/2
  Sum2/1 -> Cos1/1, Cos/1
  Cos/1 -> Product2/1
  Product2/1 -> Sum/1
  Product1/1 -> Sum1/1

== system OneAxleTrailer/Hitch/3DOF/Subsystem3/Subsystem2 ==
  Hitch Forces : Inport
  psi : Inport  Port=2
  Hitch Angles : Inport  Port=3
  Cos : Trigonometry  Operator=cos
  Cos1 : Trigonometry
  Gain : Gain  Gain=-1
  Product1 : Product
  Product2 : Product
  Sum : Sum  Inputs=+
  Sum1 : Sum  Inputs=+
  Sum2 : Sum  Inputs=|++
  Fx : Outport
  Fy : Outport  Port=2
  wires:
  Sum1/1 -> Fx/1
  Sum/1 -> Fy/1
  Product1/1 -> Sum1/1
  Product2/1 -> Sum/1
  Cos/1 -> Product2/1
  Sum2/1 -> Cos/1, Cos1/1
  psi/1 -> Sum2/2
  Hitch Forces/1 -> Gain/1
  Hitch Angles/1 -> Sum2/1
  Cos1/1 -> Product1/1
  Gain/1 -> Product1/2, Product2/2

== system OneAxleTrailer/Hitch/3DOF/Subsystem3/Trailer Hitch Contact Moment ==
  Vehicle Psi : Inport
  Trailer Psi : Inport  Port=2
  Constant : Constant  Value=0  SampleTime=-1
  Hitch Contact Yaw Moment : Lookup_n-D  NumberOfTableDimensions=1  LookupTableObject=''  BreakpointsForDimension1=[-1 -.9 -45*pi/180 0 45*pi/180 .9 1]  BreakpointsForDimension1FirstPoint=10  BreakpointsForDimension2FirstPoint=10  BreakpointsForDimension1Spacing=12  BreakpointsForDimension2Spacing=12  IndexSearchMethod=Linear search  Table=[-1e6 -1e6 0 0 0 1e6 1e6]  ExtrapMethod=Clip  DiagnosticForOutOfRangeInput=Error  UseLastTableValue=on  InternalRulePriority=Speed  RndMeth=Simplest
  Subtract : Sum  Inputs=+-
  Vector Concatenate1 : Concatenate  NumInputs=3
  Mh : Outport
  wires:
  Vector Concatenate1/1 -> Mh/1
  Constant/1 -> Vector Concatenate1/1, Vector Concatenate1/2
  Hitch Contact Yaw Moment/1 -> Vector Concatenate1/3
  Vehicle Psi/1 -> Subtract/1
  Subtract/1 -> Hitch Contact Yaw Moment/1
  Trailer Psi/1 -> Subtract/2

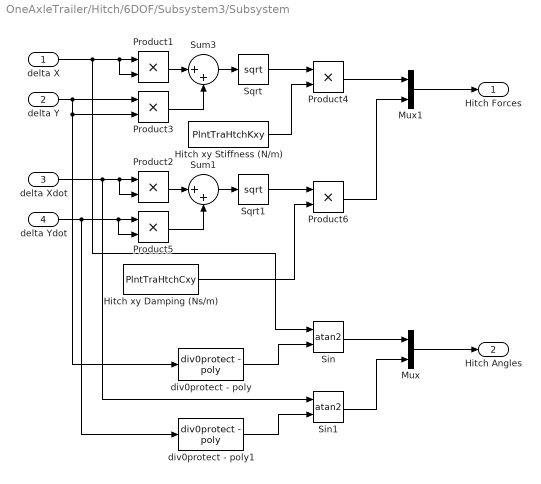
== system OneAxleTrailer/Hitch/6DOF/Subsystem3/Subsystem ==
  delta X : Inport
  delta Y : Inport  Port=2
  delta Xdot : Inport  Port=3
  delta Ydot : Inport  Port=4
  Hitch xy Damping (Ns/m) : Constant  Value=PlntTraHtchCxy  SampleTime=-1
  Hitch xy Stiffness (N/m) : Constant  Value=PlntTraHtchKxy  SampleTime=-1
  Mux : Mux  Inputs=2
  Mux1 : Mux  Inputs=2
  Product{1..6} (6 alike) : Product
  Sin : Trigonometry  Operator=atan2
  Sin1 : Trigonometry  Operator=atan2
  Sqrt : Sqrt
  Sqrt1 : Sqrt
  Sum1 : Sum  Inputs=|++
  Sum3 : Sum  Inputs=|++
  div0protect - poly : autolibutils/div0protect - poly  thresh=eps  ZeroCross=off  ZeroCross1=off  aMode=2
  div0protect - poly1 : autolibutils/div0protect - poly  thresh=eps  ZeroCross=off  ZeroCross1=off  aMode=2
  Hitch Forces : Outport
  Hitch Angles : Outport  Port=2
  wires:
  Product6/1 -> Mux1/2
  Mux1/1 -> Hitch Forces/1
  Sin1/1 -> Mux/2
  div0protect - poly1/1 -> Sin1/2
  Mux/1 -> Hitch Angles/1
  delta Ydot/1 -> Product5/2, Product5/1, div0protect - poly1/1
  Hitch xy Damping (Ns/m)/1 -> Product6/2
  delta Xdot/1 -> Product2/1, Product2/2, Sin1/1
  Sum1/1 -> Sqrt1/1
  Product2/1 -> Sum1/1
  Product5/1 -> Sum1/2
  Sqrt1/1 -> Product6/1
  Hitch xy Stiffness (N/m)/1 -> Product4/2
  Product4/1 -> Mux1/1
  Sqrt/1 -> Product4/1
  Product3/1 -> Sum3/2
  Product1/1 -> Sum3/1
  Sum3/1 -> Sqrt/1
  delta Y/1 -> div0protect - poly/1, Product3/2, Product3/1
  delta X/1 -> Product1/2, Product1/1, Sin/1
  Sin/1 -> Mux/1
  div0protect - poly/1 -> Sin/2

== system OneAxleTrailer/Hitch/6DOF/Subsystem3/Subsystem1 ==
  Hitch Forces : Inport
  psi : Inport  Port=2
  Hitch Angles : Inport  Port=3
  Cos : Trigonometry  Operator=cos
  Cos1 : Trigonometry
  Product1 : Product
  Product2 : Product
  Sum : Sum  Inputs=+
  Sum1 : Sum  Inputs=+
  Sum2 : Sum  Inputs=|++
  Fx : Outport
  Fy : Outport  Port=2
  wires:
  Sum1/1 -> Fx/1
  Sum/1 -> Fy/1
  Product1/1 -> Sum1/1
  Product2/1 -> Sum/1
  Cos/1 -> Product2/1
  Sum2/1 -> Cos/1, Cos1/1
  psi/1 -> Sum2/2
  Hitch Forces/1 -> Product1/2, Product2/2
  Hitch Angles/1 -> Sum2/1
  Cos1/1 -> Product1/1

== system OneAxleTrailer/Hitch/6DOF/Subsystem3/Subsystem2 ==
  Hitch Forces : Inport
  psi : Inport  Port=2
  Hitch Angles : Inport  Port=3
  Cos : Trigonometry  Operator=cos
  Cos1 : Trigonometry
  Gain : Gain  Gain=-1
  Product1 : Product
  Product2 : Product
  Sum : Sum  Inputs=+
  Sum1 : Sum  Inputs=+
  Sum2 : Sum  Inputs=|++
  Fx : Outport
  Fy : Outport  Port=2
  wires:
  Sum1/1 -> Fx/1
  Sum/1 -> Fy/1
  Gain/1 -> Product2/2, Product1/2
  Cos1/1 -> Product1/1
  Hitch Angles/1 -> Sum2/1
  Hitch Forces/1 -> Gain/1
  psi/1 -> Sum2/2
  Sum2/1 -> Cos1/1, Cos/1
  Cos/1 -> Product2/1
  Product2/1 -> Sum/1
  Product1/1 -> Sum1/1

== system OneAxleTrailer/Hitch/6DOF/Subsystem3/Subsystem3 ==
  Vehicle Z : Inport
  Trailer Z : Inport  Port=2
  Vehicle Zdot : Inport  Port=3
  Trailer Zdot : Inport  Port=4
  Constant8 : Constant  Value=PlntTraHtchF0z  SampleTime=-1
  Gain5 : Gain  Gain=PlntTraHtchKz
  Gain6 : Gain  Gain=PlntTraHtchCz
  Sum1 : Sum  Inputs=|--
  Sum2 : Sum  Inputs=|+-
  Sum3 : Sum  Inputs=|+-
  Sum4 : Sum  Inputs=|+-
  Trailer Fz : Outport
  wires:
  Trailer Z/1 -> Sum2/1
  Sum3/1 -> Gain6/1
  Vehicle Zdot/1 -> Sum3/2
  Trailer Zdot/1 -> Sum3/1
  Sum2/1 -> Gain5/1
  Gain6/1 -> Sum1/2
  Sum1/1 -> Sum4/1
  Constant8/1 -> Sum4/2
  Gain5/1 -> Sum1/1
  Sum4/1 -> Trailer Fz/1
  Vehicle Z/1 -> Sum2/2
